simulink model "RCAM_Simulation"  (Simulink 7.7)
settings: Solver=ode45  StartTime=0.0  StopTime=TF  RelTol=1e-3
values from neighbouring files (symbols this model uses):
  u1max = 25*pi/180    (= 0.436332312999)    [InitializationConstant.m]
  u1min = -25*pi/180    (= -0.436332312999)    [InitializationConstant.m]
  u2max = 10*pi/180    (= 0.174532925199)    [InitializationConstant.m]
  u2min = -25*pi/180    (= -0.436332312999)    [InitializationConstant.m]
  u3max = 30*pi/180    (= 0.523598775598)    [InitializationConstant.m]
  u3min = -30*pi/180    (= -0.523598775598)    [InitializationConstant.m]
  u4max = 10*pi/180    (= 0.174532925199)    [InitializationConstant.m]
  u4min = 0.5*pi/180    (= 0.00872664625997)    [InitializationConstant.m]
  u5max = 10*pi/180    (= 0.174532925199)    [InitializationConstant.m]
  u5min = 0.5*pi/180    (= 0.00872664625997)    [InitializationConstant.m]
  x0 = [85 ... (first row only)    [InitializationConstant.m]
undefined symbols (not defined in the file or in its folder): RCAM_model
settings Model: Creator=Harsha S  LastModifiedBy=Harsha S
settings DebuggingCC: SolverPrmCheckMsg=none

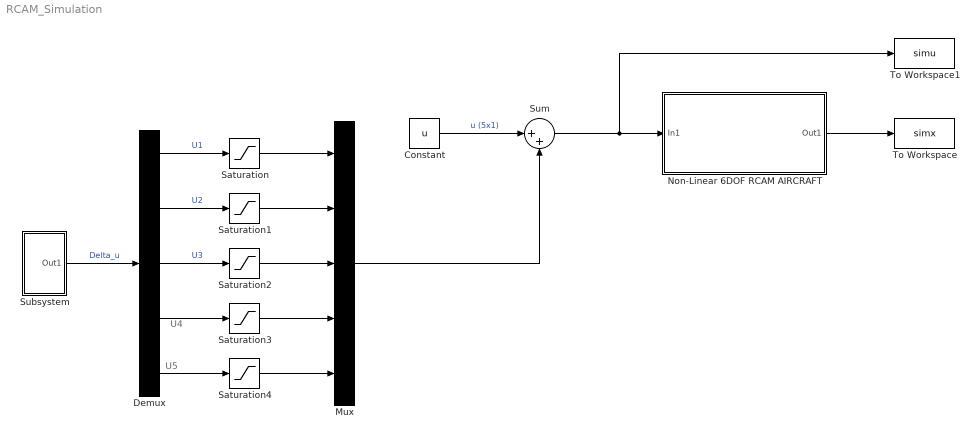
== system RCAM_Simulation ==
  note: U4
  note: U5
  Constant : Constant  Value=u
  Demux : Demux  Outputs=5
  Mux : Mux  Inputs=5
  "Non-Linear 6DOF RCAM AIRCRAFT " : Subsystem
  Saturation : Saturate  UpperLimit=u1max  LowerLimit=u1min
  Saturation1 : Saturate  UpperLimit=u2max  LowerLimit=u2min
  Saturation2 : Saturate  UpperLimit=u3max  LowerLimit=u3min
  Saturation3 : Saturate  UpperLimit=u4max  LowerLimit=u4min
  Saturation4 : Saturate  UpperLimit=u5max  LowerLimit=u5min
  Subsystem : Subsystem
  Sum : Sum  Inputs=|++
  To Workspace : ToWorkspace  VariableName=simx  SampleTime=-1  SaveFormat=Structure With Time
  To Workspace1 : ToWorkspace  VariableName=simu  SampleTime=-1  SaveFormat=Structure With Time
  wires:
  Constant/1 -> Sum/1  "u (5x1)"
  Sum/1 -> "Non-Linear 6DOF RCAM AIRCRAFT "/1(In1), To Workspace1/1
  Subsystem/1(Out1) -> Demux/1  "Delta_u"
  Demux/1 -> Saturation/1  "U1"
  Demux/2 -> Saturation1/1  "U2"
  Demux/3 -> Saturation2/1  "U3"
  Demux/4 -> Saturation3/1
  Demux/5 -> Saturation4/1
  Saturation/1 -> Mux/1
  Saturation1/1 -> Mux/2
  Saturation2/1 -> Mux/3
  Saturation3/1 -> Mux/4
  Saturation4/1 -> Mux/5
  Mux/1 -> Sum/2
  "Non-Linear 6DOF RCAM AIRCRAFT "/1(Out1) -> To Workspace/1

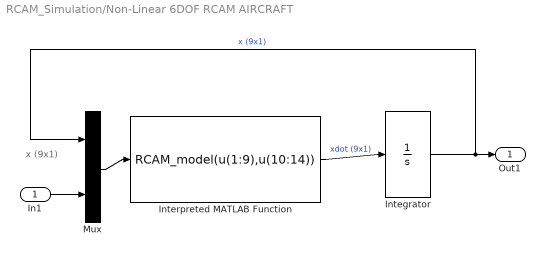
== system RCAM_Simulation/Non-Linear 6DOF RCAM AIRCRAFT  ==
  note: x (9x1)
  In1 : Inport
  Integrator : Integrator  InitialCondition=x0
  Interpreted MATLAB Function : MATLABFcn  MATLABFcn=RCAM_model(u(1:9),u(10:14))
  Mux : Mux  Inputs=2
  Out1 : Outport
  wires:
  Interpreted MATLAB Function/1 -> Integrator/1  "xdot (9x1)"
  Mux/1 -> Interpreted MATLAB Function/1
  Integrator/1 -> Mux/1, Out1/1  "x (9x1)"
  In1/1 -> Mux/2

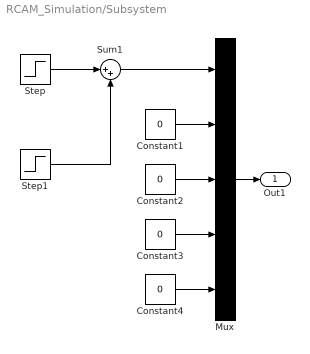
== system RCAM_Simulation/Subsystem ==
  Constant{1..4} (4 alike) : Constant  Value=0
  Mux : Mux  Inputs=5
  Step : Step  Time=30  After=5*pi/180  SampleTime=0
  Step1 : Step  Time=30+2  After=-5*pi/180  SampleTime=0
  Sum1 : Sum  Inputs=|++
  Out1 : Outport
  wires:
  Step/1 -> Sum1/1
  Step1/1 -> Sum1/2
  Sum1/1 -> Mux/1
  Constant1/1 -> Mux/2
  Constant2/1 -> Mux/3
  Constant3/1 -> Mux/4
  Constant4/1 -> Mux/5
  Mux/1 -> Out1/1
